simulink model "Subsystem1"  (R2020a)
settings: Solver=VariableStepAuto  StartTime=0.0  StopTime=10.0  RelTol=1e-3
settings Model: Creator=DELL  LastModifiedBy=DELL
settings DataIOCC: SaveOutput=off  SaveTime=off

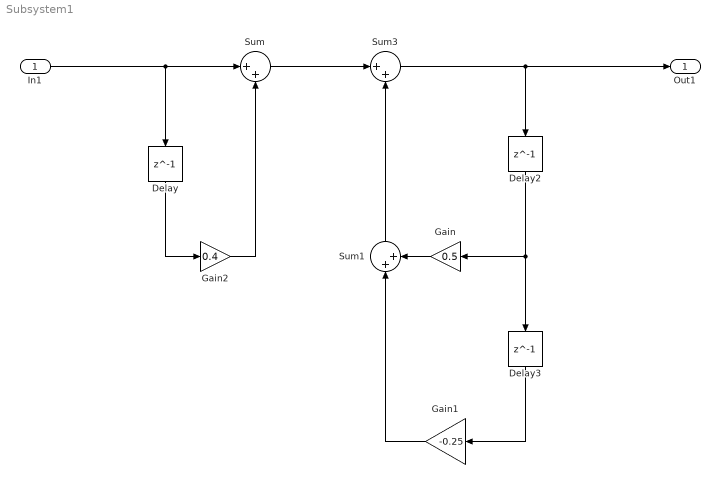
== system Subsystem1 ==
  In1 : Inport  OutDataTypeStr=double  PortDimensions=1  SampleTime=[0,1]
  Delay : Delay  DelayLength=1
  Delay2 : Delay  DelayLength=1
  Delay3 : Delay  DelayLength=1
  Gain : Gain  Gain=0.5
  Gain1 : Gain  Gain=-0.25
  Gain2 : Gain  Gain=0.4
  Sum : Sum  Inputs=|++
  Sum1 : Sum  Inputs=|++
  Sum3 : Sum  Inputs=|++
  Out1 : Outport  OutDataTypeStr=double  PortDimensions=1  SampleTime=[0,1]
  wires:
  Delay3/1 -> Gain1/1
  In1/1 -> Delay/1, Sum/1
  Delay2/1 -> Gain/1, Delay3/1
  Gain1/1 -> Sum1/1
  Delay/1 -> Gain2/1
  Gain2/1 -> Sum/2
  Sum1/1 -> Sum3/2
  Gain/1 -> Sum1/2
  Sum/1 -> Sum3/1
  Sum3/1 -> Delay2/1, Out1/1
